simulink subsystem "BtnDebounce"  (R2022a)
settings: Solver=VariableStepAuto  StartTime=0.0  StopTime=10.0  RelTol=1e-3
libraries: simulink x1
settings Model: Creator=bkfre  LastModifiedBy=bkfre

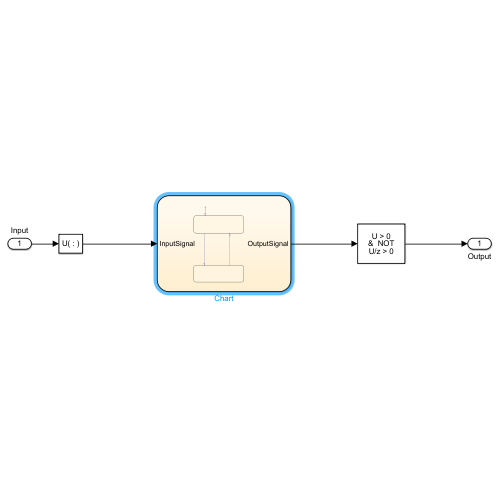
[thumbnail: Simulink's stored preview of the top-level diagram]
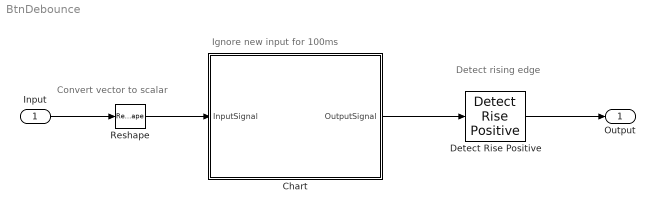
== system BtnDebounce ==
  note: Convert vector to scalar
  note: Ignore new input for 100ms
  note: Detect rising edge
  Input : Inport
  Chart : Stateflow chart  TreatAsAtomicUnit=on
  Detect Rise Positive : simulink/Logic and Bit Operations/Detect Rise Positive  vinit=0  OutDataTypeStr=boolean
  Reshape : Reshape
  Output : Outport
  wires:
  Input/1 -> Reshape/1
  Reshape/1 -> Chart/1(InputSignal)
  Detect Rise Positive/1 -> Output/1
  Chart/1(OutputSignal) -> Detect Rise Positive/1

== stateflow chart BtnDebounce/Chart ==
  state Idle
    entry:
    OutputSignal=0;
  state High
    entry:
    OutputSignal=1;
  (default) -> Idle
  Idle -> High : [duration(InputSignal>0,msec)>0.2]
  High -> Idle : [duration(InputSignal<=0,msec)>0.2]
  data: InputSignal input boolean; OutputSignal output int8
